simulink library "HDL_ieee_8021513"  (R2024a)
settings: Solver=FixedStepDiscrete  StartTime=0.0  StopTime=10.0  RelTol=1e-3
undefined symbols (not defined in the file): Add, axiWidth, CONST, fs, peakDetectorThreshold, peakDetectorWindow, QAM, Shift
libraries: hdlsllib x199, $bdroot x91, whdlutilities x34, whdledac x9, simulink x8, whdlmod x6, dspsigops x5, dsphdlfiltering2 x4, embreciprocals x3, dsphdlsigops2 x2, commhdlcrc x2, dspstat3 x2
(part 3 of 6)

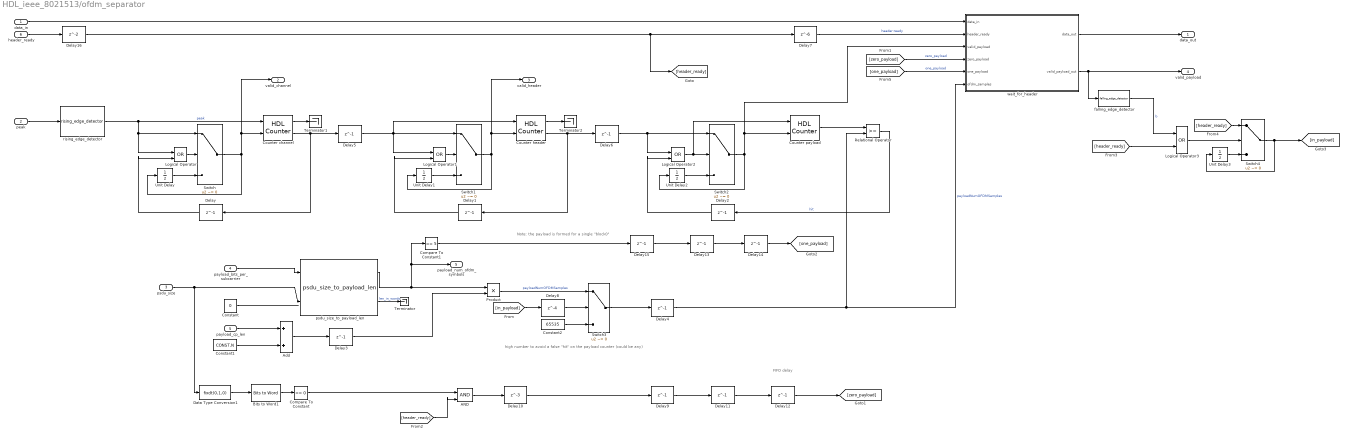
== system HDL_ieee_8021513/ofdm_separator ==
  note: FIFO delay
  note: Note: the payload is formed for a single "block0"
  note: high number to avoid a false "hit" on the payload counter (could be any)
  data_in : Inport
  peak : Inport  Port=2
  psdu_size : Inport  Port=3
  payload_bits_per_subcarrier : Inport  Port=4
  payload_cp_len : Inport  Port=5
  header_ready : Inport  Port=6
  AND : Logic  IconShape=distinctive  AllPortsSameDT=off  OutDataTypeStr=boolean
  Add : Sum  OutDataTypeStr=fixdt(0,16,0)
  Bits to Word1 : hdlsllib/Logic and Bit Operations/Bits to Word
  Compare To Constant : hdlsllib/Logic and Bit Operations/Compare To Constant  relop===  const=0  OutDataTypeStr=boolean
  Compare To Constant1 : hdlsllib/Logic and Bit Operations/Compare To Constant  relop===  const=5  OutDataTypeStr=boolean
  Constant : Constant  Value=0  OutDataTypeStr=boolean  SampleTime=1/CONST.fPHY
  Constant1 : Constant  Value=CONST.N  OutDataTypeStr=fixdt(0,9,0)  SampleTime=-1
  Constant2 : Constant  Value=65535  OutDataTypeStr=Inherit: Inherit via back propagation  SampleTime=-1
  Counter channel : hdlsllib/Sources/HDL Counter  CountType=Count limited  CountInit=0  CountStep=1  CountMax=CONST.channelOFDMSamples-2  CountFromType=Initial value  CountFrom=0  CountResetPort=on  CountLoadPort=off  CountEnbPort=on  CountDirPort=off  CountHitOutputPort=on  CountDataType=Unsigned  CountWordLen=nextpow2(CONST.channelOFDMSamples)  CountFracLen=0  CountSampTime=1
  Counter header : hdlsllib/Sources/HDL Counter  CountType=Count limited  CountInit=0  CountStep=1  CountMax=CONST.headerOFDMSamples-2  CountFromType=Initial value  CountFrom=0  CountResetPort=on  CountLoadPort=off  CountEnbPort=on  CountDirPort=off  CountHitOutputPort=on  CountDataType=Unsigned  CountWordLen=nextpow2(CONST.headerOFDMSamples)  CountFracLen=0  CountSampTime=1
  Counter payload : hdlsllib/Sources/HDL Counter  CountType=Free running  CountInit=2  CountStep=1  CountMax=1  CountFromType=Initial value  CountFrom=2  CountResetPort=on  CountLoadPort=off  CountEnbPort=on  CountDirPort=off  CountHitOutputPort=off  CountDataType=Unsigned  CountWordLen=32  CountFracLen=0  CountSampTime=1
  Data Type Conversion1 : DataTypeConversion  OutDataTypeStr=fixdt(0,1,0)  SaturateOnIntegerOverflow=off  RndMeth=Floor
  Delay{,1..6,9,11..15} (13 alike) : Delay  DelayLength=1  InitialCondition=0  UseCircularBuffer=on
  Delay10 : Delay  DelayLength=3  InitialCondition=0  UseCircularBuffer=on
  Delay16 : Delay  InitialCondition=0  UseCircularBuffer=on
  Delay7 : Delay  DelayLength=6  InitialCondition=0  UseCircularBuffer=on
  Delay8 : Delay  DelayLength=4  InitialCondition=0  UseCircularBuffer=on
  Logical Operator{,1..3} (4 alike) : Logic  Operator=OR  IconShape=distinctive  AllPortsSameDT=off  OutDataTypeStr=boolean
  Product : Product
  Relational Operator : RelationalOperator  OutDataTypeStr=boolean  InputSameDT=off
  Switch{,1..2,4} (4 alike) : Switch  Criteria=u2 ~= 0  SaturateOnIntegerOverflow=off  InputSameDT=off
  Switch3 : Switch  Criteria=u2 ~= 0  SaturateOnIntegerOverflow=off
  Terminator : Terminator
  Terminator1 : Terminator
  Terminator2 : Terminator
  Unit Delay{,1..3} (4 alike) : UnitDelay  SampleTime=-1  HasFrameUpgradeWarning=on
  falling_edge_detector : $bdroot/falling_edge_detector  SystemSampleTime=-1  VariantActivationTime=update diagram  AllowFlexibleInterface=on  Latency=0  AutoFrameSizeCalculation=off
  psdu_size_to_payload_len : $bdroot/payload_full/psdu_size_to_payload_len  SystemSampleTime=-1  VariantActivationTime=update diagram  AllowFlexibleInterface=on  Latency=0  AutoFrameSizeCalculation=off
  rising_edge_detector : $bdroot/rising_edge_detector  SystemSampleTime=-1  VariantActivationTime=update diagram  AllowFlexibleInterface=on  Latency=0  AutoFrameSizeCalculation=off
  wait_for_header : Subsystem
  data_out : Outport  VectorParamsAs1DForOutWhenUnconnected=off
  valid_channel : Outport  Port=2
  valid_header : Outport  Port=3
  valid_payload : Outport  Port=4
  payload_num_ofdm_symbols : Outport  Port=5  VectorParamsAs1DForOutWhenUnconnected=off
  wires:
  psdu_size_to_payload_len/2 -> Terminator/1  "len_in_words"
  Delay16/1 -> [header_ready], Delay7/1
  peak/1 -> rising_edge_detector/1
  Counter channel/1 -> Terminator1/1
  Counter header/1 -> Terminator2/1
  Unit Delay/1 -> Switch/3
  Switch/1 -> valid_channel/1, Counter channel/2, Unit Delay/1
  Logical Operator/1 -> Switch/2
  Counter channel/2 -> Delay5/1, Delay/1
  Delay/1 -> Logical Operator/2
  Delay1/1 -> Logical Operator1/2
  Logical Operator1/1 -> Switch1/2
  Unit Delay1/1 -> Switch1/3
  Switch1/1 -> Unit Delay1/1, valid_header/1, Counter header/2
  Delay2/1 -> Logical Operator2/2
  Unit Delay2/1 -> Switch2/3
  Logical Operator2/1 -> Counter payload/1, Switch2/2
  Switch2/1 -> wait_for_header/3(valid_payload), Counter payload/2, Unit Delay2/1
  Counter header/2 -> Delay6/1, Delay1/1
  rising_edge_detector/1 -> Logical Operator/1, Switch/1, Counter channel/1  "peak"
  Constant1/1 -> Add/2
  payload_cp_len/1 -> Add/1
  Add/1 -> Delay3/1
  Relational Operator/1 -> Delay2/1  "hit"
  Counter payload/1 -> Relational Operator/1
  Delay5/1 -> Counter header/1, Logical Operator1/1, Switch1/1
  psdu_size/1 -> Data Type Conversion1/1, psdu_size_to_payload_len/2
  payload_bits_per_subcarrier/1 -> psdu_size_to_payload_len/1
  Constant/1 -> ?
  psdu_size_to_payload_len/1 -> Compare To Constant1/1, payload_num_ofdm_symbols/1, Product/1
  Delay3/1 -> Product/2
  data_in/1 -> wait_for_header/1(data_in)
  wait_for_header/1(data_out) -> data_out/1
  wait_for_header/2(valid_payload_out) -> valid_payload/1, falling_edge_detector/1
  Product/1 -> Switch3/1  "payloadNumOFDMSamples"
  Constant2/1 -> Switch3/3
  Switch3/1 -> Delay4/1
  Delay4/1 -> wait_for_header/6(ofdm_samples), Relational Operator/2  "payloadNumOFDMSamples"
  header_ready/1 -> Delay16/1
  Data Type Conversion1/1 -> Bits to Word1/1
  Bits to Word1/1 -> Compare To Constant/1
  [zero_payload] -> wait_for_header/4(zero_payload)  "zero_payload"
  [header_ready] -> AND/2
  AND/1 -> Delay10/1
  [in_payload] -> Delay8/1
  falling_edge_detector/1 -> Logical Operator3/1  "b"
  Delay6/1 -> Switch2/1, Logical Operator2/1
  Unit Delay3/1 -> Switch4/3
  Switch4/1 -> Unit Delay3/1, [in_payload]
  Logical Operator3/1 -> Switch4/2
  [header_ready] -> Logical Operator3/2
  [header_ready] -> Switch4/1
  Delay7/1 -> wait_for_header/2(header_ready)  "header:ready"
  Delay8/1 -> Switch3/2
  Delay9/1 -> Delay11/1
  [one_payload] -> wait_for_header/5(one_payload)  "one_payload"
  Compare To Constant/1 -> AND/1
  Delay11/1 -> Delay12/1
  Delay12/1 -> [zero_payload]
  Delay15/1 -> Delay13/1
  Compare To Constant1/1 -> Delay15/1
  Delay10/1 -> Delay9/1
  Delay13/1 -> Delay14/1
  Delay14/1 -> [one_payload]

== system HDL_ieee_8021513/ofdm_symbol_sync ==
  note: peakSync is synchronized with the first element of the channel
  note: Delay of find_peak = peakDetectorWindow
  data_in : Inport
  Delay : Delay  DelayLength=CONST.preambleOFDMSamples-20  InitialCondition=0  UseCircularBuffer=on
  Delay1 : Delay  DelayLength=128  InitialCondition=0  UseCircularBuffer=on
  Delay2 : Delay  DelayLength=20  InitialCondition=0  UseCircularBuffer=on
  find_peak : Subsystem
  m_cox : Subsystem
  phase_offset_calculator : Subsystem
  data_out : Outport
  peak_sync : Outport  Port=2
  phase_offset : Outport  Port=3  VectorParamsAs1DForOutWhenUnconnected=off
  M(d) : Outport  Port=4
  reset_ofdm : Outport  Port=5  VectorParamsAs1DForOutWhenUnconnected=off
  wires:
  Delay2/1 -> peak_sync/1
  data_in/1 -> m_cox/1(data_in)
  m_cox/2(M(d)) -> find_peak/2(M_in), M(d)/1
  m_cox/3(P(d)) -> Delay1/1
  m_cox/1(data_out) -> find_peak/1(data_in)
  find_peak/1(data_out) -> data_out/1
  find_peak/2(peak_sync) -> Delay/1, phase_offset_calculator/1(peak_sync)
  Delay/1 -> Delay2/1, reset_ofdm/1
  Delay1/1 -> phase_offset_calculator/2(P(d))
  phase_offset_calculator/1(frequency_offset) -> phase_offset/1

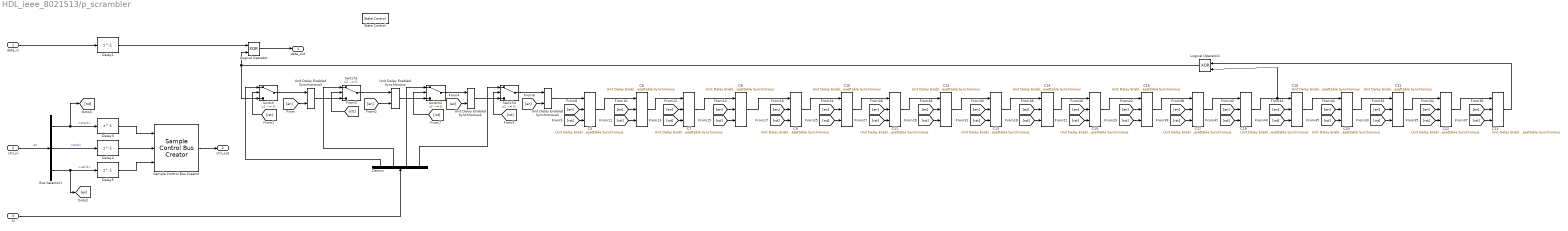
== system HDL_ieee_8021513/p_scrambler ==
  data_in : Inport
  ctrl_in : Inport  Port=2
  SI : Inport  Port=3
  Bus Selector1 : BusSelector  OutputSignals=start,end,valid
  C{5..23} (19 alike) : hdlsllib/Discrete/Unit Delay Enabled Resettable Synchronous  InitialCondition=1  SampleTime=-1
  Delay{1,3..5} (4 alike) : Delay  DelayLength=1  InitialCondition=0  UseCircularBuffer=on
  Demux : Demux
  Logical Operator : Logic  Operator=XOR  IconShape=distinctive  AllPortsSameDT=off  OutDataTypeStr=boolean
  Logical Operator1 : Logic  Operator=XOR  IconShape=distinctive  AllPortsSameDT=off  OutDataTypeStr=boolean
  Sample Control Bus Creator : whdlutilities/Sample Control Bus Creator
  State Control : StateControl  StateControl=Synchronous
  Switch{,1..3} (4 alike) : Switch  Criteria=u2 ~= 0  OutDataTypeStr=boolean  SaturateOnIntegerOverflow=off  InputSameDT=off
  Unit Delay Enabled Synchronous{,1..3} (4 alike) : hdlsllib/Discrete/Unit Delay Enabled Synchronous  InitialCondition=1  SampleTime=-1
  data_out : Outport
  ctrl_out : Outport  Port=2  VectorParamsAs1DForOutWhenUnconnected=off
  wires:
  Logical Operator1/1 -> Switch/3, Logical Operator/2
  Logical Operator/1 -> data_out/1
  ctrl_in/1 -> Bus Selector1/1  "en"
  data_in/1 -> Delay1/1
  Delay1/1 -> Logical Operator/1
  SI/1 -> Demux/1
  Demux/2 -> Switch1/1
  [en] -> Unit Delay Enabled Synchronous3/2
  [en] -> Unit Delay Enabled Synchronous/2
  [en] -> Unit Delay Enabled Synchronous1/2
  [en] -> Unit Delay Enabled Synchronous2/2
  [en] -> C5/2
  [en] -> C7/2
  [rst] -> C8/3
  C7/1 -> C8/1
  [rst] -> C7/3
  C5/1 -> C6/1
  [rst] -> C6/3
  [en] -> C8/2
  C6/1 -> C7/1
  [en] -> C6/2
  [rst] -> C5/3
  Unit Delay Enabled Synchronous2/1 -> C5/1
  C15/1 -> C16/1
  C9/1 -> C10/1
  [rst] -> C12/3
  [en] -> C16/2
  [rst] -> C11/3
  [en] -> C13/2
  C12/1 -> C13/1
  [rst] -> C10/3
  C10/1 -> C11/1
  [rst] -> C13/3
  [en] -> C11/2
  C14/1 -> C15/1
  [en] -> C9/2
  [en] -> C10/2
  [rst] -> C9/3
  C11/1 -> C12/1
  C13/1 -> C14/1
  [rst] -> C14/3
  [en] -> C12/2
  [rst] -> C16/3
  [en] -> C14/2
  [en] -> C15/2
  [rst] -> C15/3
  C8/1 -> C9/1
  [rst] -> C17/3
  [rst] -> C23/3
  C16/1 -> C17/1
  [en] -> C22/2
  C20/1 -> C21/1
  C18/1 -> Logical Operator1/2, C19/1
  [rst] -> C20/3
  [en] -> C23/2
  [en] -> C18/2
  [en] -> C19/2
  C22/1 -> C23/1
  C17/1 -> C18/1
  [rst] -> C21/3
  [rst] -> C19/3
  [en] -> C17/2
  [rst] -> C18/3
  C21/1 -> C22/1
  [en] -> C21/2
  [en] -> C20/2
  C19/1 -> C20/1
  [rst] -> C22/3
  C23/1 -> Logical Operator1/1
  [rst] -> Switch/2
  Demux/1 -> Switch/1
  Switch/1 -> Unit Delay Enabled Synchronous3/1
  Switch1/1 -> Unit Delay Enabled Synchronous/1
  [rst] -> Switch1/2
  Unit Delay Enabled Synchronous3/1 -> Switch1/3
  Switch2/1 -> Unit Delay Enabled Synchronous1/1
  Switch3/1 -> Unit Delay Enabled Synchronous2/1
  Unit Delay Enabled Synchronous1/1 -> Switch3/3
  [rst] -> Switch3/2
  Demux/4 -> Switch3/1
  Demux/3 -> Switch2/1
  Unit Delay Enabled Synchronous/1 -> Switch2/3
  [rst] -> Switch2/2
  Bus Selector1/1 -> [rst], Delay3/1  "<start>"
  Bus Selector1/2 -> Delay4/1  "<end>"
  Bus Selector1/3 -> [en], Delay5/1  "<valid>"
  Delay3/1 -> Sample Control Bus Creator/1
  Delay4/1 -> Sample Control Bus Creator/2
  Delay5/1 -> Sample Control Bus Creator/3
  Sample Control Bus Creator/1 -> ctrl_out/1

== system HDL_ieee_8021513/payload_full ==
  note: Note: careful when adding delays to signals "ready, valid or data" outside this block
  data_in : Inport
  valid_in : Inport  Port=2
  new_frame : Inport  Port=3
  scrambler_init : Inport  Port=4
  bat_id : Inport  Port=5
  psdu_size : Inport  Port=6
  Delay{,1..12} (13 alike) : Delay  DelayLength=1  InitialCondition=0  UseCircularBuffer=on
  Delay13 : Delay  DelayLength=8  InitialCondition=0  UseCircularBuffer=on
  HDL Counter : hdlsllib/Sources/HDL Counter  CountType=Free running  CountInit=0  CountStep=1  CountMax=25  CountFromType=Initial value  CountFrom=0  CountResetPort=on  CountLoadPort=off  CountEnbPort=on  CountDirPort=off  CountHitOutputPort=off  CountDataType=Unsigned  CountWordLen=32  CountFracLen=0  CountSampTime=1
  HDL FIFO : hdlsllib/HDL RAMs/HDL FIFO  fifo_size=5000  mode=Classic  ratio=1  push_msg=Error  pop_msg=Error  show_empty=off  show_full=on  show_num=off  LabelModeActiveChoice_Mode=Classic  rst_port=off
  Logical Operator1 : Logic  IconShape=distinctive  AllPortsSameDT=off  OutDataTypeStr=boolean
  Logical Operator5 : Logic  Operator=OR  IconShape=distinctive  AllPortsSameDT=off  OutDataTypeStr=boolean
  NOT : Logic  Operator=NOT  IconShape=distinctive  AllPortsSameDT=off  OutDataTypeStr=boolean
  Rate Transition : RateTransition  OutPortSampleTimeOpt=Multiple of input port sample time  OutPortSampleTimeMultiple=8  OutPortSampleTime=1/fs
  Rate Transition1 : RateTransition  OutPortSampleTimeOpt=Multiple of input port sample time  OutPortSampleTimeMultiple=1/8
  Rate Transition4 : RateTransition  OutPortSampleTimeOpt=Multiple of input port sample time  OutPortSampleTimeMultiple=1/8
  Rate Transition5 : RateTransition  OutPortSampleTimeOpt=Multiple of input port sample time  OutPortSampleTimeMultiple=1/8  OutPortSampleTime=1/axiWidth
  Rate Transition6 : RateTransition  OutPortSampleTimeOpt=Multiple of input port sample time  OutPortSampleTimeMultiple=1/8
  Relational Operator : RelationalOperator  OutDataTypeStr=boolean  InputSameDT=off
  Serializer1D : hdlsllib/HDL Operations/Serializer1D  Ratio=8  IdleCycles=0  validIn=on  startOut=off  validOut=on  inputDataDimensions=-1  inputSampleTime=-1  inputSignalType=auto
  State Control : StateControl  StateControl=Synchronous
  Switch1 : Switch  Criteria=u2 ~= 0  SaturateOnIntegerOverflow=off  InputSameDT=off
  Unit Delay1 : UnitDelay  SampleTime=-1  HasFrameUpgradeWarning=on
  Word to Bits : hdlsllib/Logic and Bit Operations/Word to Bits  maxWordLength=8
  batid_to_bits_per_subcarrier : $bdroot/batid_to_bits_per_subcarrier  SystemSampleTime=-1  VariantActivationTime=update diagram  AllowFlexibleInterface=on  Latency=0  AutoFrameSizeCalculation=off
  next_frame_to_ready : $bdroot/next_frame_to_ready  SystemSampleTime=-1  VariantActivationTime=update diagram  AllowFlexibleInterface=on  Latency=0  AutoFrameSizeCalculation=off
  p_scrambler : $bdroot/p_scrambler  SystemSampleTime=-1  VariantActivationTime=update diagram  AllowFlexibleInterface=on  Latency=0  AutoFrameSizeCalculation=off
      settings: LibrarySourceBlock=|
      | hdlsllib/Ports &
      | Subsystems/Subsystem
  psdu_size_to_payload_length : $bdroot/psdu_size_to_payload_length  SystemSampleTime=-1  VariantActivationTime=update diagram  AllowFlexibleInterface=on  Latency=0  AutoFrameSizeCalculation=off
  reduced_ldpc : $bdroot/reduced_ldpc  SystemSampleTime=-1  VariantActivationTime=update diagram  AllowFlexibleInterface=on  Latency=0  AutoFrameSizeCalculation=off
  rising_edge_detector : $bdroot/rising_edge_detector  SystemSampleTime=-1  VariantActivationTime=update diagram  AllowFlexibleInterface=on  Latency=0  AutoFrameSizeCalculation=off
  tone_mapping : $bdroot/tone_mapping  SystemSampleTime=-1  VariantActivationTime=update diagram  AllowFlexibleInterface=on  Latency=0  AutoFrameSizeCalculation=off
  valid_to_ctrl : $bdroot/valid_to_ctrl  SystemSampleTime=-1  VariantActivationTime=update diagram  AllowFlexibleInterface=on  Latency=0  AutoFrameSizeCalculation=off
  payload : Outport  VectorParamsAs1DForOutWhenUnconnected=off
  ctrl_out : Outport  Port=2  VectorParamsAs1DForOutWhenUnconnected=off
  ready : Outport  Port=3  VectorParamsAs1DForOutWhenUnconnected=off
  len_in_ofdm_symbols : Outport  Port=4  VectorParamsAs1DForOutWhenUnconnected=off
  bits_per_subcarrier : Outport  Port=5  VectorParamsAs1DForOutWhenUnconnected=off
  wires:
  Delay13/1 -> HDL FIFO/3, Delay2/1  "pop"
  HDL FIFO/1 -> Word to Bits/1
  Delay4/1 -> HDL FIFO/1
  Delay3/1 -> HDL FIFO/2
  Delay12/1 -> ready/1
  NOT/1 -> Delay12/1
  HDL FIFO/2 -> NOT/1
  valid_in/1 -> Delay3/1
  data_in/1 -> Delay4/1
  Delay11/1 -> [new_frame]
  Delay10/1 -> tone_mapping/4, len_in_ofdm_symbols/1
  Delay6/1 -> tone_mapping/3, bits_per_subcarrier/1
  Delay9/1 -> p_scrambler/3
  Delay8/1 -> p_scrambler/2
  Delay7/1 -> p_scrambler/1
  Rate Transition1/1 -> Delay9/1
  [last_frame] -> Logical Operator5/2
  [word_valid] -> HDL Counter/2
  psdu_size_to_payload_length/2 -> Relational Operator/2  "len_in_words"
  [new_frame_slow] -> HDL Counter/1
  rising_edge_detector/1 -> [last_frame]  "last_frame"
  Relational Operator/1 -> rising_edge_detector/1
  HDL Counter/1 -> Relational Operator/1  "counter"
  [new_frame] -> tone_mapping/5
  Rate Transition6/1 -> Delay11/1
  Rate Transition5/1 -> Delay10/1  "len_in_ofdm_symbols"
  Rate Transition4/1 -> Delay6/1  "bits_per_subcarrier"
  psdu_size_to_payload_length/1 -> Rate Transition5/1
  psdu_size/1 -> psdu_size_to_payload_length/2
  bat_id/1 -> batid_to_bits_per_subcarrier/1
  batid_to_bits_per_subcarrier/1 -> Rate Transition4/1, psdu_size_to_payload_length/1
  tone_mapping/1 -> payload/1
  reduced_ldpc/2 -> tone_mapping/2  "ctrl_in"
  tone_mapping/2 -> ctrl_out/1
  new_frame/1 -> Logical Operator5/1, Switch1/1, Rate Transition6/1, [new_frame_slow]
  Logical Operator5/1 -> Switch1/2
  Switch1/1 -> Unit Delay1/1, Logical Operator1/1
  Unit Delay1/1 -> Switch1/3
  Logical Operator1/1 -> next_frame_to_ready/1
  Rate Transition/1 -> Delay5/1
  Delay2/1 -> Serializer1D/2, [word_valid]
  next_frame_to_ready/1 -> Delay13/1  "ready"
  reduced_ldpc/3 -> Delay1/1
  Delay1/1 -> Rate Transition/1
  Word to Bits/1 -> Serializer1D/1
  Serializer1D/1 -> Delay/1
  Serializer1D/2 -> valid_to_ctrl/1
  valid_to_ctrl/1 -> Delay8/1
  Delay/1 -> Delay7/1
  reduced_ldpc/1 -> tone_mapping/1  "dataOut"
  scrambler_init/1 -> Rate Transition1/1
  p_scrambler/1 -> reduced_ldpc/1
  p_scrambler/2 -> reduced_ldpc/2
  Delay5/1 -> Logical Operator1/2

== system HDL_ieee_8021513/payload_rep ==
  data_in : Inport
  ctrl_in : Inport  Port=2
  data_out : Outport
  ctrl_out : Outport  Port=2
  wires:
  data_in/1 -> data_out/1
  ctrl_in/1 -> ctrl_out/1

== system HDL_ieee_8021513/peak_detector ==
  note: TODO: local peak not working correctly
  note: This block has a latency of 19 clock cycles
  dataIn : Inport
  local_peak : Subsystem
  s1_index : Subsystem
  peak_sync : Outport
  wires:
  s1_index/1(indexes) -> local_peak/1(index)
  s1_index/2(Output) -> local_peak/2(dataIn)
  dataIn/1 -> s1_index/1(dataIn)
  local_peak/1(peak_sync) -> peak_sync/1

== system HDL_ieee_8021513/preamble_gen ==
  new_frame : Inport
  Delay : Delay  DelayLength=1  InitialCondition=0  UseCircularBuffer=on
  Direct Lookup Table (n-D) : LookupNDDirect  NumberOfTableDimensions=1  Table=CONST.preambleLUT  DiagnosticForOutOfRangeInput=Error  RemoveProtectionInput=on  TableDataTypeStr=boolean
  HDL Counter : hdlsllib/Sources/HDL Counter  CountType=Count limited  CountInit=0  CountStep=1  CountMax=length(CONST.preambleLUT)-1  CountFromType=Initial value  CountFrom=0  CountResetPort=off  CountLoadPort=off  CountEnbPort=on  CountDirPort=off  CountHitOutputPort=on  CountDataType=Unsigned  CountWordLen=nextpow2(length(CONST.preambleLUT))  CountFracLen=0  CountSampTime=1
  Logical Operator : Logic  Operator=NOT  IconShape=distinctive  AllPortsSameDT=off  OutDataTypeStr=boolean
  Logical Operator1 : Logic  Operator=OR  IconShape=distinctive  AllPortsSameDT=off  OutDataTypeStr=boolean
  State Control : StateControl  StateControl=Synchronous
  Unit Delay Enabled Synchronous : hdlsllib/Discrete/Unit Delay Enabled Synchronous  InitialCondition=0.0  SampleTime=-1
  valid_to_ctrl : $bdroot/valid_to_ctrl  SystemSampleTime=-1  VariantActivationTime=update diagram  AllowFlexibleInterface=on  Latency=0  AutoFrameSizeCalculation=off
  data_out : Outport
  ctrl_out : Outport  Port=2
  wires:
  HDL Counter/1 -> Direct Lookup Table (n-D)/1
  Logical Operator/1 -> Unit Delay Enabled Synchronous/1
  HDL Counter/2 -> Logical Operator/1, Logical Operator1/2
  Logical Operator1/1 -> Unit Delay Enabled Synchronous/2
  new_frame/1 -> Logical Operator1/1
  Direct Lookup Table (n-D)/1 -> Delay/1
  Unit Delay Enabled Synchronous/1 -> valid_to_ctrl/1, HDL Counter/1
  valid_to_ctrl/1 -> ctrl_out/1
  Delay/1 -> data_out/1

== system HDL_ieee_8021513/psdu_size_to_payload_length ==
  note: Get length of the payload expressed in OFDM Symbols:
      |
      | bitsInPsdu = psduSize * 8 * fecRate [bits/payload]
      | bitsInOFDMSymbol = numDataCarriers * bitsPerSubcarrier [bits/OFDM]
      |
      | payloadLenInOFDMSymbols = ceil( bitsInPsdu / bitsInOFDMSymbol ) [OFDM/payload]
  bits_per_subcarrier : Inport
  psdu_size : Inport  Port=2
  Bit Shift : hdlsllib/Logic and Bit Operations/Bit Shift  mode=Shift Left Logical  N=4
  Bit Shift2 : hdlsllib/Logic and Bit Operations/Bit Shift  mode=Shift Right Arithmetic  N=0
  Bit Shift3 : hdlsllib/Logic and Bit Operations/Bit Shift  mode=Shift Right Arithmetic  N=1
  Bit Shift5 : hdlsllib/Logic and Bit Operations/Bit Shift  mode=Shift Right Arithmetic  N=4
  Bits to Word1 : hdlsllib/Logic and Bit Operations/Bits to Word
  Data Type Conversion1 : DataTypeConversion  OutDataTypeStr=fixdt(0,1,0)  SaturateOnIntegerOverflow=off  RndMeth=Floor
  Delay{,1..3} (4 alike) : Delay  InitialCondition=0  UseCircularBuffer=on
  Gain : Gain  Gain=fi(1/CONST.numDataCarriers, 0, 16, 16)  ParamDataTypeStr=fixdt(1,16,15)  OutDataTypeStr=uint16  RndMeth=Ceiling
  Multiport Switch : MultiPortSwitch  DataPortOrder=Zero-based contiguous  Inputs=5  zeroidx=on  SaturateOnIntegerOverflow=off  InputSameDT=off
  State Control : StateControl  StateControl=Synchronous
  payload_len_in_ofdm_symbols : Outport
  payload_len_in_words : Outport  Port=2  VectorParamsAs1DForOutWhenUnconnected=off
  wires:
  Gain/1 -> Delay2/1
  Delay1/1 -> Multiport Switch/1
  Delay/1 -> Bit Shift3/1, Bit Shift5/1, Bit Shift2/1
  Bit Shift5/1 -> Multiport Switch/6
  Bit Shift3/1 -> Multiport Switch/4, Multiport Switch/5
  Bit Shift2/1 -> Multiport Switch/3, Multiport Switch/2
  Bit Shift/1 -> Delay/1
  Delay2/1 -> payload_len_in_ofdm_symbols/1
  Bits to Word1/1 -> Bit Shift/1, payload_len_in_words/1
  psdu_size/1 -> Data Type Conversion1/1
  Multiport Switch/1 -> Delay3/1
  Data Type Conversion1/1 -> Bits to Word1/1
  bits_per_subcarrier/1 -> Delay1/1
  Delay3/1 -> Gain/1

== system HDL_ieee_8021513/puncturer ==
  data_in : Inport
  ctrl_in : Inport  Port=2
  data_out : Outport
  ctrl_out : Outport  Port=2
  wires:
  data_in/1 -> data_out/1
  ctrl_in/1 -> ctrl_out/1

== system HDL_ieee_8021513/qam_demod ==
  note: Note: using not a defailt QAM constellation results in an error while doing the HDL Code Generation
  data_in : Inport
  valid_in : Inport  Port=2
  bits_per_subcarrier : Inport  Port=3
  Constant{1..2,4..5} (4 alike) : Constant  Value=[0; 0; 0; 0]  VectorParams1D=off  OutDataTypeStr=Inherit: Inherit via back propagation  SampleTime=-1  LockScale=on
  Data Type Conversion3 : DataTypeConversion  OutDataTypeStr=fixdt(1,16,10)  SaturateOnIntegerOverflow=off  RndMeth=Floor
  Delay : Delay  DelayLength=1  InitialCondition=0  UseCircularBuffer=on
  Delay1 : Delay  DelayLength=1  InitialCondition=0  UseCircularBuffer=on
  Delay2 : Delay  DelayLength=0  InitialCondition=0  UseCircularBuffer=on
  Delay3 : Delay  DelayLength=1  InitialCondition=0  UseCircularBuffer=on
  Delay4 : Delay  DelayLength=0  InitialCondition=0  UseCircularBuffer=on
  Delay5 : Delay  DelayLength=6  InitialCondition=0  UseCircularBuffer=on
  Delay7 : Delay  DelayLength=6  InitialCondition=0  UseCircularBuffer=on
  Multiport Switch : MultiPortSwitch  DataPortOrder=Zero-based contiguous  Inputs=8  zeroidx=on  OutDataTypeStr=Inherit: Same as first data input  SaturateOnIntegerOverflow=off
  Symbol Demodulator : whdlmod/Symbol Demodulator  ModulationSource=Property  ModulationScheme=BPSK  MaxModulation=256-QAM  ConstOrder=Default  ConstMap=[ 2, 3, 1, 0, 6, 7, 5, 4, 14, 15, 13, 12, 10, 11, 9, 8 ]  DecisionType=Approximate log-likelihood ratio  PhaseOffset=0  OutputType=Vector  NormMethod=Unit average power  MinSymDistance=2  NoiseVariance=off  SimulateUsing=Code generation
  Symbol Demodulator1 : whdlmod/Symbol Demodulator  ModulationSource=Property  ModulationScheme=QPSK  MaxModulation=256-QAM  ConstOrder=Default  ConstMap=[ 2, 3, 1, 0, 6, 7, 5, 4, 14, 15, 13, 12, 10, 11, 9, 8 ]  DecisionType=Approximate log-likelihood ratio  PhaseOffset=-pi/4  OutputType=Vector  NormMethod=Unit average power  MinSymDistance=2  NoiseVariance=off  SimulateUsing=Code generation
  Symbol Demodulator2 : whdlmod/Symbol Demodulator  ModulationSource=Property  ModulationScheme=16-QAM  MaxModulation=256-QAM  ConstOrder=Default  ConstMap=qamFourBits.'  DecisionType=Approximate log-likelihood ratio  PhaseOffset=pi/2  OutputType=Vector  NormMethod=Unit average power  MinSymDistance=2  NoiseVariance=off  SimulateUsing=Code generation
  Terminator : Terminator
  Terminator1 : Terminator
  Terminator2 : Terminator
  to_12bit_integer : Subsystem
  data_out : Outport
  valid_out : Outport  Port=2  VectorParamsAs1DForOutWhenUnconnected=off
  wires:
  Data Type Conversion3/1 -> data_out/1
  Delay/1 -> Data Type Conversion3/1
  to_12bit_integer/1(1bit_out) -> Multiport Switch/3, Multiport Switch/2
  Constant1/1 -> Multiport Switch/7
  bits_per_subcarrier/1 -> Delay7/1
  Delay1/1 -> valid_out/1
  Constant2/1 -> Multiport Switch/5
  Constant5/1 -> Multiport Switch/9
  valid_in/1 -> Delay5/1, Symbol Demodulator/2, Symbol Demodulator1/2, Symbol Demodulator2/2
  Multiport Switch/1 -> Delay/1
  Delay7/1 -> Multiport Switch/1
  Constant4/1 -> Multiport Switch/8
  data_in/1 -> Symbol Demodulator2/1, Symbol Demodulator1/1, Symbol Demodulator/1
  Symbol Demodulator/1 -> Delay2/1
  Symbol Demodulator1/1 -> Delay3/1
  Symbol Demodulator2/1 -> Delay4/1
  Symbol Demodulator2/2 -> Terminator/1
  Symbol Demodulator/2 -> Terminator1/1
  Symbol Demodulator1/2 -> Terminator2/1
  Delay5/1 -> Delay1/1
  Delay2/1 -> to_12bit_integer/1(1bit)
  Delay3/1 -> to_12bit_integer/2(2bit)
  Delay4/1 -> to_12bit_integer/3(4bit)
  to_12bit_integer/3(4bit_out) -> Multiport Switch/6
  to_12bit_integer/2(2bit_out) -> Multiport Switch/4

== system HDL_ieee_8021513/qam_mod ==
  data_in : Inport
  valid_in : Inport  Port=2
  bits_per_subcarrier : Inport  Port=3
  BPSK Modulator Baseband : commdigbbndpm3/BPSK Modulator Baseband  Ph=0  outDtype=Fixed-point  outWordLen=16  outUDDataType=sfix(16)  outFracLenMode=User-defined  outFracLen=14  outDataTypeStr=fixdt(1,16,14)  outLastDataTypeStr=fixdt(1,16,14)
      settings: LibrarySourceBlock=|
      | commhdldigbbndpm/BPSK
      | Modulator
      | Baseband
  Bit Slice : hdlsllib/Logic and Bit Operations/Bit Slice  lidx=0  ridx=0
  Bit Slice1 : hdlsllib/Logic and Bit Operations/Bit Slice  lidx=1  ridx=0
  Constant{2..5} (4 alike) : Constant  Value=0  OutDataTypeStr=Inherit: Inherit via back propagation  SampleTime=-1  LockScale=on
  Delay : Delay  DelayLength=1  InitialCondition=0  UseCircularBuffer=on
  Delay1 : Delay  DelayLength=1  InitialCondition=0  UseCircularBuffer=on
  Multiport Switch : MultiPortSwitch  DataPortOrder=Zero-based contiguous  Inputs=4  zeroidx=on  SaturateOnIntegerOverflow=off
  Real-Imag to Complex1 : RealImagToComplex
  Real-Imag to Complex2 : RealImagToComplex
  State Control : StateControl  StateControl=Synchronous
  batID 1 : commdigbbndam3/Rectangular QAM Modulator Baseband  M=4  InType=Integer  Enc=User-defined  Mapping=CONST.qamTwoBits  PowType=Average Power  MinDist=2  AvgPow=1  PeakPow=1  Ph=0  outDtype=Fixed-point  outWordLen=16  outUDDataType=sfix(16)  outFracLenMode=User-defined  outFracLen=14  outDataTypeStr=fixdt(1,16,14)  outLastDataTypeStr=fixdt(1,16,14)
      settings: LibrarySourceBlock=|
      | commhdldigbbndam/Rectangular QAM
      | Modulator
      | Baseband
  data_out : Outport
  valid_out : Outport  Port=2  VectorParamsAs1DForOutWhenUnconnected=off
  wires:
  valid_in/1 -> Delay1/1
  Delay1/1 -> valid_out/1
  data_in/1 -> Bit Slice1/1, Bit Slice/1
  bits_per_subcarrier/1 -> Multiport Switch/1
  Multiport Switch/1 -> Delay/1
  Bit Slice/1 -> BPSK Modulator Baseband/1
  Bit Slice1/1 -> batID 1/1
  batID 1/1 -> Multiport Switch/4
  Real-Imag to Complex2/1 -> Multiport Switch/5
  Delay/1 -> data_out/1
  BPSK Modulator Baseband/1 -> Multiport Switch/3
  Constant3/1 -> Real-Imag to Complex1/1
  Real-Imag to Complex1/1 -> Multiport Switch/2
  Constant5/1 -> Real-Imag to Complex1/2
  Constant4/1 -> Real-Imag to Complex2/2
  Constant2/1 -> Real-Imag to Complex2/1

== system HDL_ieee_8021513/reduced_ldpc ==
  data_in : Inport
  ctrl_in : Inport  Port=2
  Delay{,1..4} (5 alike) : Delay  DelayLength=1  InitialCondition=0  UseCircularBuffer=on
  Hc_12S-B80 : whdledac/LDPC Encoder  ParityCheckMatrix=CONST.Hc_12H  BlockSize=14  SimulateUsing=Code generation
  State Control : StateControl  StateControl=Synchronous
  data_out : Outport
  ctrl_out : Outport  Port=2
  next_frame : Outport  Port=3
  wires:
  Delay4/1 -> next_frame/1
  Delay3/1 -> ctrl_out/1
  Delay2/1 -> data_out/1
  Delay1/1 -> Hc_12S-B80/2
  Delay/1 -> Hc_12S-B80/1
  ctrl_in/1 -> Delay1/1
  Hc_12S-B80/3 -> Delay4/1
  data_in/1 -> Delay/1
  Hc_12S-B80/1 -> Delay2/1
  Hc_12S-B80/2 -> Delay3/1

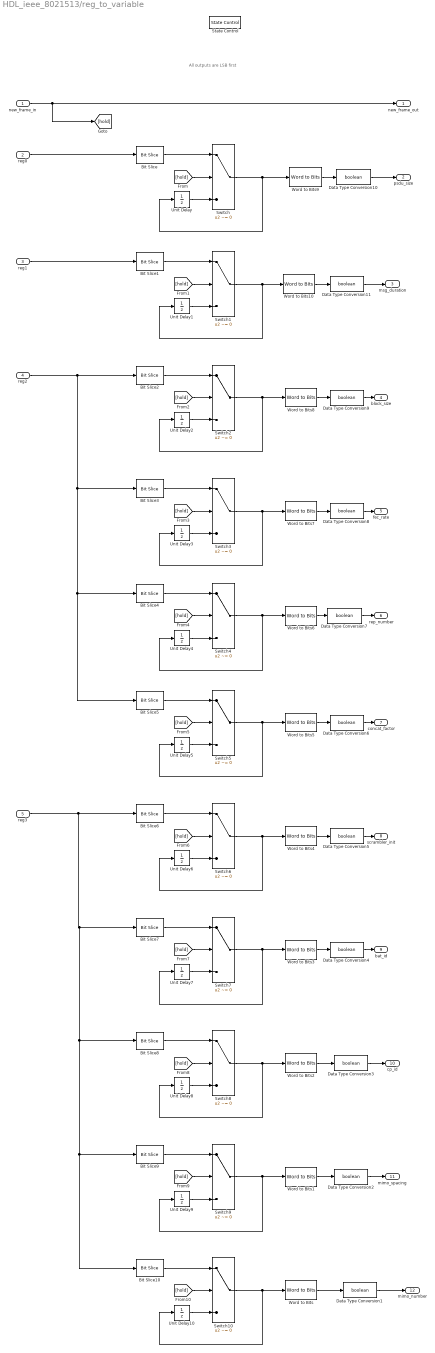
== system HDL_ieee_8021513/reg_to_variable ==
  note: All outputs are LSB first
  new_frame_in : Inport
  reg0 : Inport  Port=2
  reg1 : Inport  Port=3
  reg2 : Inport  Port=4
  reg3 : Inport  Port=5
  Bit Slice : hdlsllib/Logic and Bit Operations/Bit Slice  lidx=23  ridx=0
  Bit Slice1 : hdlsllib/Logic and Bit Operations/Bit Slice  lidx=15  ridx=0
  Bit Slice10 : hdlsllib/Logic and Bit Operations/Bit Slice  lidx=29  ridx=27
  Bit Slice2 : hdlsllib/Logic and Bit Operations/Bit Slice  lidx=1  ridx=0
  Bit Slice3 : hdlsllib/Logic and Bit Operations/Bit Slice  lidx=10  ridx=8
  Bit Slice4 : hdlsllib/Logic and Bit Operations/Bit Slice  lidx=18  ridx=16
  Bit Slice5 : hdlsllib/Logic and Bit Operations/Bit Slice  lidx=26  ridx=24
  Bit Slice6 : hdlsllib/Logic and Bit Operations/Bit Slice  lidx=3  ridx=0
  Bit Slice7 : hdlsllib/Logic and Bit Operations/Bit Slice  lidx=12  ridx=8
  Bit Slice8 : hdlsllib/Logic and Bit Operations/Bit Slice  lidx=18  ridx=16
  Bit Slice9 : hdlsllib/Logic and Bit Operations/Bit Slice  lidx=26  ridx=24
  Data Type Conversion{1..11} (11 alike) : DataTypeConversion  OutDataTypeStr=boolean  SaturateOnIntegerOverflow=off  RndMeth=Floor
  State Control : StateControl  StateControl=Synchronous
  Switch{,1..10} (11 alike) : Switch  Criteria=u2 ~= 0  SaturateOnIntegerOverflow=off  InputSameDT=off
  Unit Delay{,1..10} (11 alike) : UnitDelay  SampleTime=-1  HasFrameUpgradeWarning=on
  Word to Bits{,1..2,5..7} (6 alike) : hdlsllib/Logic and Bit Operations/Word to Bits  maxWordLength=3
  Word to Bits10 : hdlsllib/Logic and Bit Operations/Word to Bits  maxWordLength=16
  Word to Bits3 : hdlsllib/Logic and Bit Operations/Word to Bits  maxWordLength=5
  Word to Bits4 : hdlsllib/Logic and Bit Operations/Word to Bits  maxWordLength=4
  Word to Bits8 : hdlsllib/Logic and Bit Operations/Word to Bits  maxWordLength=2
  Word to Bits9 : hdlsllib/Logic and Bit Operations/Word to Bits  maxWordLength=24
  new_frame_out : Outport  VectorParamsAs1DForOutWhenUnconnected=off
  psdu_size : Outport  Port=2  VectorParamsAs1DForOutWhenUnconnected=off
  msg_duration : Outport  Port=3  VectorParamsAs1DForOutWhenUnconnected=off
  block_size : Outport  Port=4  VectorParamsAs1DForOutWhenUnconnected=off
  fec_rate : Outport  Port=5  VectorParamsAs1DForOutWhenUnconnected=off
  rep_number : Outport  Port=6  VectorParamsAs1DForOutWhenUnconnected=off
  concat_factor : Outport  Port=7  VectorParamsAs1DForOutWhenUnconnected=off
  scrambler_init : Outport  Port=8  VectorParamsAs1DForOutWhenUnconnected=off
  bat_id : Outport  Port=9  VectorParamsAs1DForOutWhenUnconnected=off
  cp_id : Outport  Port=10  VectorParamsAs1DForOutWhenUnconnected=off
  mimo_spacing : Outport  Port=11  VectorParamsAs1DForOutWhenUnconnected=off
  mimo_number : Outport  Port=12  VectorParamsAs1DForOutWhenUnconnected=off
  wires:
  reg3/1 -> Bit Slice10/1, Bit Slice9/1, Bit Slice8/1, Bit Slice7/1, Bit Slice6/1
  reg2/1 -> Bit Slice5/1, Bit Slice4/1, Bit Slice3/1, Bit Slice2/1
  Bit Slice/1 -> Switch/1
  reg1/1 -> Bit Slice1/1
  Unit Delay/1 -> Switch/3
  [hold] -> Switch/2
  reg0/1 -> Bit Slice/1
  Bit Slice1/1 -> Switch1/1
  Unit Delay1/1 -> Switch1/3
  [hold] -> Switch1/2
  [hold] -> Switch2/2
  Unit Delay2/1 -> Switch2/3
  Bit Slice2/1 -> Switch2/1
  Switch2/1 -> Word to Bits8/1, Unit Delay2/1
  Bit Slice3/1 -> Switch3/1
  Switch3/1 -> Word to Bits7/1, Unit Delay3/1
  Unit Delay3/1 -> Switch3/3
  [hold] -> Switch3/2
  Bit Slice6/1 -> Switch6/1
  Bit Slice7/1 -> Switch7/1
  Unit Delay7/1 -> Switch7/3
  Switch5/1 -> Word to Bits5/1, Unit Delay5/1
  Bit Slice5/1 -> Switch5/1
  Switch6/1 -> Word to Bits4/1, Unit Delay6/1
  Unit Delay5/1 -> Switch5/3
  [hold] -> Switch7/2
  Bit Slice4/1 -> Switch4/1
  [hold] -> Switch5/2
  Unit Delay6/1 -> Switch6/3
  Unit Delay4/1 -> Switch4/3
  Switch4/1 -> Word to Bits6/1, Unit Delay4/1
  [hold] -> Switch4/2
  Switch7/1 -> Word to Bits3/1, Unit Delay7/1
  [hold] -> Switch6/2
  Unit Delay9/1 -> Switch9/3
  Bit Slice9/1 -> Switch9/1
  [hold] -> Switch9/2
  [hold] -> Switch8/2
  [hold] -> Switch10/2
  Switch9/1 -> Word to Bits1/1, Unit Delay9/1
  Unit Delay8/1 -> Switch8/3
  Bit Slice8/1 -> Switch8/1
  Bit Slice10/1 -> Switch10/1
  Switch8/1 -> Word to Bits2/1, Unit Delay8/1
  Unit Delay10/1 -> Switch10/3
  Switch10/1 -> Word to Bits/1, Unit Delay10/1
  new_frame_in/1 -> new_frame_out/1, [hold]
  Word to Bits/1 -> Data Type Conversion1/1
  Word to Bits1/1 -> Data Type Conversion2/1
  Word to Bits2/1 -> Data Type Conversion3/1
  Word to Bits3/1 -> Data Type Conversion4/1
  Word to Bits4/1 -> Data Type Conversion5/1
  Word to Bits5/1 -> Data Type Conversion6/1
  Word to Bits6/1 -> Data Type Conversion7/1
  Word to Bits8/1 -> Data Type Conversion9/1
  Word to Bits7/1 -> Data Type Conversion8/1
  Data Type Conversion1/1 -> mimo_number/1
  Data Type Conversion2/1 -> mimo_spacing/1
  Data Type Conversion3/1 -> cp_id/1
  Data Type Conversion4/1 -> bat_id/1
  Data Type Conversion5/1 -> scrambler_init/1
  Data Type Conversion6/1 -> concat_factor/1
  Data Type Conversion7/1 -> rep_number/1
  Data Type Conversion8/1 -> fec_rate/1
  Data Type Conversion9/1 -> block_size/1
  Switch1/1 -> Word to Bits10/1, Unit Delay1/1
  Switch/1 -> Word to Bits9/1, Unit Delay/1
  Word to Bits9/1 -> Data Type Conversion10/1
  Data Type Conversion10/1 -> psdu_size/1
  Word to Bits10/1 -> Data Type Conversion11/1
  Data Type Conversion11/1 -> msg_duration/1

== system HDL_ieee_8021513/remove_tone_mapping ==
  data_in : Inport
  valid_in : Inport  Port=2
  newFrame : Inport  Port=3
  psdu_size : Inport  Port=4
  Bits to Word : hdlsllib/Logic and Bit Operations/Bits to Word
  Data Type Conversion : DataTypeConversion  OutDataTypeStr=fixdt(0,1,0)  SaturateOnIntegerOverflow=off  RndMeth=Floor
  Delay : Delay  DelayLength=1  InitialCondition=0  UseCircularBuffer=on
  HDL Counter : hdlsllib/Sources/HDL Counter  CountType=Free running  CountInit=0  CountStep=1  CountMax=25  CountFromType=Initial value  CountFrom=0  CountResetPort=on  CountLoadPort=off  CountEnbPort=on  CountDirPort=off  CountHitOutputPort=off  CountDataType=Unsigned  CountWordLen=32  CountFracLen=0  CountSampTime=1
  Logical Operator : Logic  IconShape=distinctive  AllPortsSameDT=off  OutDataTypeStr=boolean
  Multiply by 2 (for fec_rate 1/2) : hdlsllib/Logic and Bit Operations/Bit Shift  mode=Shift Left Logical  N=1
  Multiply by 8 : hdlsllib/Logic and Bit Operations/Bit Shift  mode=Shift Left Logical  N=3
  Relational Operator : RelationalOperator  Operator=<  OutDataTypeStr=boolean  InputSameDT=off
  valid_to_ctrl : $bdroot/valid_to_ctrl  SystemSampleTime=-1  VariantActivationTime=update diagram  AllowFlexibleInterface=on  Latency=0  AutoFrameSizeCalculation=off
  data_out : Outport
  ctrl_out : Outport  Port=2
  wires:
  newFrame/1 -> HDL Counter/1
  Multiply by 2 (for fec_rate 1/2)/1 -> Relational Operator/2
  Delay/1 -> data_out/1
  valid_to_ctrl/1 -> ctrl_out/1
  psdu_size/1 -> Data Type Conversion/1
  Bits to Word/1 -> Multiply by 8/1
  HDL Counter/1 -> Relational Operator/1  "Count"
  Multiply by 8/1 -> Multiply by 2 (for fec_rate 1/2)/1
  Logical Operator/1 -> valid_to_ctrl/1  "valid_out"
  Relational Operator/1 -> Logical Operator/2
  Data Type Conversion/1 -> Bits to Word/1
  valid_in/1 -> HDL Counter/2, Logical Operator/1
  data_in/1 -> Delay/1

== system HDL_ieee_8021513/rising_edge_detector ==
  In : Inport
  Delay2 : Delay  DelayLength=1  InitialCondition=0  UseCircularBuffer=on
  Logical Operator1 : Logic  IconShape=distinctive  AllPortsSameDT=off  OutDataTypeStr=boolean
  Logical Operator2 : Logic  Operator=NOT  IconShape=distinctive  AllPortsSameDT=off  OutDataTypeStr=boolean
  State Control : StateControl  StateControl=Synchronous
  Out : Outport
  wires:
  Logical Operator2/1 -> Logical Operator1/2
  Delay2/1 -> Logical Operator2/1
  In/1 -> Logical Operator1/1, Delay2/1
  Logical Operator1/1 -> Out/1

== system HDL_ieee_8021513/rx_demodulator_full ==
  note: Last frame has one less delay because of the falling edge
  data_in : Inport
  payload_cp_len : Inport  Port=2
  payload_bits_per_subcarrier : Inport  Port=3
  psdu_size : Inport  Port=4
  header_ready : Inport  Port=5
  4QAM_demod : $bdroot/4QAM_demod  SystemSampleTime=-1  VariantActivationTime=update diagram  AllowFlexibleInterface=on  Latency=0  AutoFrameSizeCalculation=off
  AND1 : Logic  IconShape=distinctive  AllPortsSameDT=off  OutDataTypeStr=boolean
  AND2 : Logic  IconShape=distinctive  AllPortsSameDT=off  OutDataTypeStr=boolean
  Constant1 : Constant  OutDataTypeStr=boolean  SampleTime=-1
  Data Type Conversion : DataTypeConversion  OutDataTypeStr=CONST.rxDemodInputDataType  SaturateOnIntegerOverflow=off  RndMeth=Floor
  Data Type Conversion1 : DataTypeConversion  OutDataTypeStr=CONST.rxDecimatorOutputDataType  SaturateOnIntegerOverflow=off  RndMeth=Floor
  Delay{,2,5..6} (4 alike) : Delay  DelayLength=1  InitialCondition=0  UseCircularBuffer=on
  Delay1 : Delay  DelayLength=3  InitialCondition=0  UseCircularBuffer=on
  Delay15 : Delay  DelayLength=3  InitialCondition=0  UseCircularBuffer=on
  Delay16 : Delay  InitialCondition=0  UseCircularBuffer=on
  Delay17 : Delay  DelayLength=100  InitialCondition=0  UseCircularBuffer=on
  Delay18 : Delay  DelayLength=7  InitialCondition=0  UseCircularBuffer=on
  Delay19 : Delay  DelayLength=7  InitialCondition=0  UseCircularBuffer=on
  Delay20 : Delay  DelayLength=7  InitialCondition=0  UseCircularBuffer=on
  Delay4 : Delay  DelayLength=100  InitialCondition=0  UseCircularBuffer=on
  Delay7 : Delay  DelayLength=100  InitialCondition=0  UseCircularBuffer=on
  Delay8 : Delay  DelayLength=3  InitialCondition=0  UseCircularBuffer=on
  Logical Operator : Logic  IconShape=distinctive  AllPortsSameDT=off  OutDataTypeStr=boolean
  Logical Operator1 : Logic  Operator=OR  Inputs=3  IconShape=distinctive  AllPortsSameDT=off  OutDataTypeStr=boolean
  Logical Operator6 : Logic  IconShape=distinctive  AllPortsSameDT=off  OutDataTypeStr=boolean
  Logical Operator7 : Logic  IconShape=distinctive  AllPortsSameDT=off  OutDataTypeStr=boolean
  OR : Logic  Operator=OR  IconShape=distinctive  AllPortsSameDT=off  OutDataTypeStr=boolean
  Rate Transition : RateTransition  OutPortSampleTime=1/CONST.fDAC
  Terminator : Terminator
  Terminator1 : Terminator
  Terminator2 : Terminator
  channel_estimation_and_equalization : $bdroot/channel_estimation_and_equalization  SystemSampleTime=-1  VariantActivationTime=update diagram  AllowFlexibleInterface=on  Latency=0  AutoFrameSizeCalculation=off
  constellation_descrambler : $bdroot/constellation_descrambler  SystemSampleTime=-1  VariantActivationTime=update diagram  AllowFlexibleInterface=on  Latency=0  AutoFrameSizeCalculation=off
  decimator : $bdroot/decimator  SystemSampleTime=-1  VariantActivationTime=update diagram  AllowFlexibleInterface=on  Latency=0  AutoFrameSizeCalculation=off
  downshifter : $bdroot/downshifter  SystemSampleTime=-1  VariantActivationTime=update diagram  AllowFlexibleInterface=on  Latency=0  AutoFrameSizeCalculation=off
  get_bits_per_subcarrier : Subsystem
  get_cp : Subsystem
  get_init : Subsystem
  ofdm_demod : $bdroot/ofdm_demod  SystemSampleTime=-1  VariantActivationTime=update diagram  AllowFlexibleInterface=on  Latency=0  AutoFrameSizeCalculation=off
  ofdm_rx_counter : Subsystem
  ofdm_separator : $bdroot/ofdm_separator  SystemSampleTime=-1  VariantActivationTime=update diagram  AllowFlexibleInterface=on  Latency=0  AutoFrameSizeCalculation=off
  ofdm_symbol_sync : $bdroot/ofdm_symbol_sync  SystemSampleTime=-1  VariantActivationTime=update diagram  AllowFlexibleInterface=on  Latency=0  AutoFrameSizeCalculation=off
  data_out : Outport  VectorParamsAs1DForOutWhenUnconnected=off
  valid_header : Outport  Port=2  VectorParamsAs1DForOutWhenUnconnected=off
  valid_payload : Outport  Port=3  VectorParamsAs1DForOutWhenUnconnected=off
  last_frame : Outport  Port=4  VectorParamsAs1DForOutWhenUnconnected=off
  wires:
  [reset] -> channel_estimation_and_equalization/4
  Data Type Conversion1/1 -> ofdm_symbol_sync/1
  Data Type Conversion/1 -> downshifter/1
  Delay2/1 -> downshifter/3
  downshifter/2 -> decimator/2  "valid_out"
  downshifter/1 -> decimator/1
  decimator/2 -> Terminator2/1
  Rate Transition/1 -> Delay2/1
  Constant1/1 -> downshifter/2
  [freq_offset] -> Rate Transition/1
  4QAM_demod/1 -> data_out/1
  Delay6/1 -> constellation_descrambler/1
  Delay5/1 -> constellation_descrambler/2  "descrambler_valid"
  Logical Operator1/1 -> Logical Operator/2
  payload_cp_len/1 -> [p_cp], ofdm_separator/5
  payload_bits_per_subcarrier/1 -> ofdm_separator/4, [p_bits]
  psdu_size/1 -> ofdm_separator/3
  ofdm_demod/1 -> Delay6/1
  Delay/1 -> Logical Operator/1
  ofdm_demod/2 -> Delay5/1, ofdm_rx_counter/1(valid)  "valid_ofdm_demod_out"
  Logical Operator/1 -> ofdm_demod/2  "ofdm_valid"
  data_in/1 -> Data Type Conversion/1
  constellation_descrambler/2 -> AND2/2, AND1/1  "qam_demod_valid"
  ofdm_demod/3 -> Delay/1
  Delay20/1 -> last_frame/1
  Logical Operator7/1 -> valid_payload/1
  Logical Operator6/1 -> valid_header/1
  4QAM_demod/2 -> Logical Operator6/1, Logical Operator7/1
  ofdm_rx_counter/4(last_frame) -> Delay16/1  "last_frame"
  Delay18/1 -> Logical Operator6/2
  Delay19/1 -> Logical Operator7/2
  decimator/1 -> Data Type Conversion1/1
  ofdm_separator/1 -> ofdm_demod/1
  ofdm_symbol_sync/2 -> ofdm_separator/2  "peak_sync"
  ofdm_symbol_sync/1 -> ofdm_separator/1
  ofdm_separator/2 -> ofdm_rx_counter/2(rst), Logical Operator1/1  "valid_channel"
  ofdm_separator/3 -> Logical Operator1/2, get_cp/1(valid_header)  "valid_header"
  ofdm_separator/5 -> ofdm_rx_counter/3(payload_num_ofdm_symbols)
  get_cp/1(ofdm_cp_len) -> ofdm_demod/3  "cp_len"
  get_init/1(descrambler_init) -> constellation_descrambler/3
  ofdm_rx_counter/2(is_header) -> get_init/1(valid_header), Delay8/1  "is_header"
  ofdm_rx_counter/3(is_payload) -> get_init/2(valid_payload), Delay15/1  "is_payload"
  get_bits_per_subcarrier/1(qam_demod_bits) -> 4QAM_demod/3
  ofdm_rx_counter/1(is_channel) -> Delay1/1  "is_channel"
  Delay8/1 -> OR/1, Delay4/1
  Delay15/1 -> OR/2, Delay7/1
  OR/1 -> AND2/1
  AND1/1 -> channel_estimation_and_equalization/3
  AND2/1 -> channel_estimation_and_equalization/2
  constellation_descrambler/1 -> channel_estimation_and_equalization/1
  channel_estimation_and_equalization/3 -> Terminator/1
  channel_estimation_and_equalization/2 -> 4QAM_demod/2
  channel_estimation_and_equalization/1 -> 4QAM_demod/1
  [p_cp] -> get_cp/3(cp_payload)
  [p_bits] -> get_bits_per_subcarrier/1(payload_bits_per_sub)
  ofdm_symbol_sync/4 -> Terminator1/1
  ofdm_symbol_sync/3 -> [freq_offset]
  Delay1/1 -> AND1/2
  Delay16/1 -> Delay17/1
  Delay4/1 -> Delay18/1, get_bits_per_subcarrier/2(valid_header)
  Delay7/1 -> Delay19/1
  Delay17/1 -> Delay20/1
  ofdm_separator/4 -> Logical Operator1/3, get_cp/2(valid_payload)  "valid_payload"
  header_ready/1 -> ofdm_separator/6
  ofdm_symbol_sync/5 -> [reset]
  [reset] -> ofdm_demod/4

== system HDL_ieee_8021513/rx_interpolator ==
  data_in : Inport
  valid_in : Inport  Port=2
  Delay{,4,6..11,14..15,18} (11 alike) : Delay  DelayLength=1  InitialCondition=0  UseCircularBuffer=on
  Delay1 : Delay  DelayLength=CONST.rxInterpolatorDelay  InitialCondition=0  UseCircularBuffer=on
  Delay16 : Delay  DelayLength=CONST.rxInterpolatorDelay*(CONST.rxL-1)  InitialCondition=0  UseCircularBuffer=on
  Delay17 : Delay  DelayLength=CONST.rxInterpolatorDelay*(CONST.rxL-1)  InitialCondition=0  UseCircularBuffer=on
  Delay2 : Delay  InitialCondition=0  UseCircularBuffer=on
  Delay3 : Delay  DelayLength=CONST.rxInterpolatorDelay  InitialCondition=0  UseCircularBuffer=on
  Delay5 : Delay  InitialCondition=0  UseCircularBuffer=on
  FIR Interpolator : dsphdlfiltering2/FIR Interpolator  Numerator=CONST.rxInterpolatorFilter.Numerator  FilterStructure=Direct form systolic  InterpolationFactor=CONST.rxL  NumCycles=CONST.rxL  SimulateUsing=Code generation  roundingMode=Floor  overflowMode=off  CoefficientsDataTypeStr=fixdt(1,16,12)  OutputDataTypeStr=fixdt(1,16,12)  ResetInputPort=off  HDLGlobalReset=on
  HDL Counter : hdlsllib/Sources/HDL Counter  CountType=Count limited  CountInit=0  CountStep=1  CountMax=CONST.rxInterpolatorDelay*(CONST.rxL-1)-1  CountFromType=Initial value  CountFrom=0  CountResetPort=on  CountLoadPort=off  CountEnbPort=on  CountDirPort=off  CountHitOutputPort=on  CountDataType=Unsigned  CountWordLen=8  CountFracLen=0  CountSampTime=1
  Logical Operator : Logic  Operator=OR  IconShape=distinctive  AllPortsSameDT=off  OutDataTypeStr=boolean
  Logical Operator1 : Logic  IconShape=distinctive  AllPortsSameDT=off  OutDataTypeStr=boolean
  Logical Operator2 : Logic  AllPortsSameDT=off  OutDataTypeStr=boolean
  Logical Operator3 : Logic  Operator=NOT  AllPortsSameDT=off  OutDataTypeStr=boolean
  Logical Operator4 : Logic  Operator=OR  AllPortsSameDT=off  OutDataTypeStr=boolean
  Switch : Switch  Criteria=u2 ~= 0  SaturateOnIntegerOverflow=off  InputSameDT=off
  Terminator : Terminator
  Terminator1 : Terminator
  Unit Delay : UnitDelay  SampleTime=-1  HasFrameUpgradeWarning=on
  Upsample : dspsigops/Upsample  FactorSource=Dialog parameter  N=CONST.rxL  Nmax=16  phase=0  RateOptions=Allow multirate processing  ic=0  mode=Unused parameter value
      settings: LibrarySourceBlock=dsphdlsupportsigops/Upsample
  Upsample1 : dspsigops/Upsample  FactorSource=Dialog parameter  N=CONST.rxL  Nmax=16  phase=0  RateOptions=Allow multirate processing  ic=0  mode=Unused parameter value
      settings: LibrarySourceBlock=dsphdlsupportsigops/Upsample
  falling_edge_detector : $bdroot/falling_edge_detector  SystemSampleTime=-1  VariantActivationTime=update diagram  AllowFlexibleInterface=on  Latency=0  AutoFrameSizeCalculation=off
  data_out : Outport  VectorParamsAs1DForOutWhenUnconnected=off
  valid_out : Outport  Port=2  VectorParamsAs1DForOutWhenUnconnected=off
  wires:
  FIR Interpolator/2 -> Logical Operator1/1, Delay1/1
  Delay4/1 -> data_out/1
  Logical Operator1/1 -> Delay8/1
  Upsample/1 -> FIR Interpolator/1
  Logical Operator/1 -> Delay2/1
  Delay3/1 -> Logical Operator/2
  Delay1/1 -> Logical Operator1/2
  FIR Interpolator/3 -> Terminator1/1
  Delay/1 -> valid_out/1
  valid_in/1 -> Logical Operator/1, Delay3/1
  Upsample1/1 -> FIR Interpolator/2
  FIR Interpolator/1 -> Delay9/1
  data_in/1 -> Delay5/1
  Delay2/1 -> Upsample1/1
  Delay5/1 -> Upsample/1
  falling_edge_detector/1 -> Delay10/1  "b"
  Delay6/1 -> Delay11/1
  Delay8/1 -> falling_edge_detector/1, Delay14/1
  Delay9/1 -> Delay6/1
  Delay11/1 -> Delay17/1
  Logical Operator2/1 -> Delay/1
  HDL Counter/2 -> Delay7/1
  HDL Counter/1 -> Terminator/1  "count"
  Unit Delay/1 -> Switch/3
  Switch/1 -> Delay18/1, HDL Counter/2, Unit Delay/1  "count_enable"
  Delay10/1 -> Logical Operator4/1, Switch/1, HDL Counter/1
  Delay16/1 -> Logical Operator2/1
  Delay17/1 -> Delay4/1
  Delay14/1 -> Delay15/1
  Delay15/1 -> Delay16/1
  Logical Operator4/1 -> Switch/2
  Delay7/1 -> Logical Operator4/2
  Logical Operator3/1 -> Logical Operator2/2
  Delay18/1 -> Logical Operator3/1
